simulink model "DCM_Test_v5"  (Simulink 7.5)
settings: Solver=FixedStepDiscrete  StartTime=0.0  StopTime=t(end)  FixedStep=SampleT  RelTol=1e-3
values from neighbouring files (symbols this model uses):
  apSampleTime = 0.01    [demoz2SlugsV5.m]
  R0 = single(Euler2DCMdeg( PHI_IC, THETA_IC, PSI_IC ))    [demoz2SlugsV5.m]
  SampleT = 0.02    [demoz2SlugsV5.m]
undefined symbols (not defined in the file or in its folder): DiscIntNeverNeededParam
libraries: simulink x11, dspmtrx3 x2
settings Model: Creator=Robert  LastModifiedBy=Robert
settings DataIOCC: LimitDataPoints=off

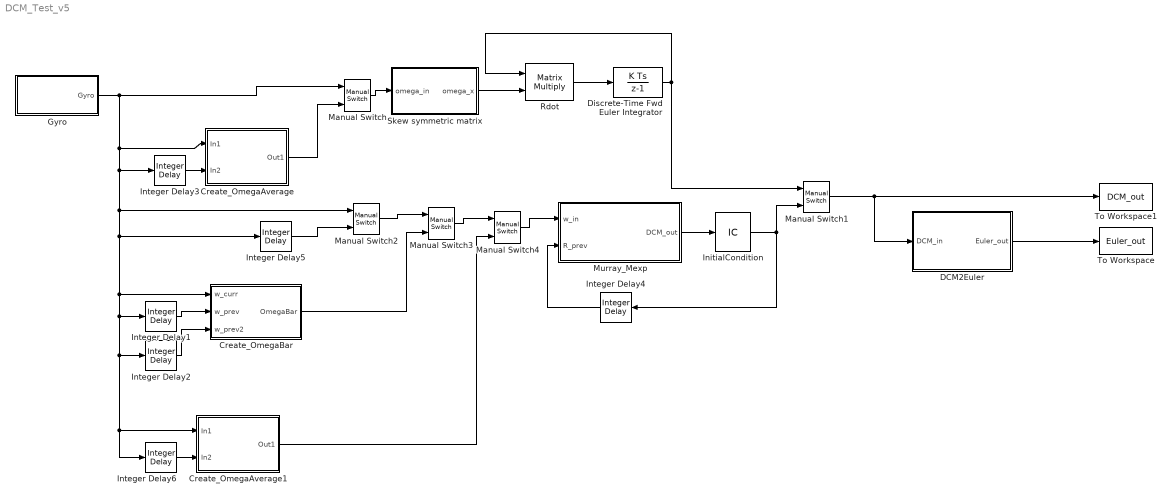
== system DCM_Test_v5 ==
  Create_OmegaAverage : Subsystem
  Create_OmegaAverage1 : Subsystem
  Create_OmegaBar : Subsystem
  DCM2Euler : Subsystem
  Discrete-Time Fwd Euler Integrator : DiscreteIntegrator  InitialCondition=R0  SampleTime=SampleT  OutDataTypeMode=single  OutDataType=fixdt(1, 16)  OutScaling=2^0  OutDataTypeStr=single  ICPrevOutput=DiscIntNeverNeededParam  ICPrevScaledInput=DiscIntNeverNeededParam
  Gyro : Subsystem
  InitialCondition : InitialCondition  Value=R0  SampleTime=apSampleTime
  Integer Delay{1,3..6} (5 alike) : simulink/Discrete/Integer Delay  vinit=0.0  samptime=-1  NumDelays=1
  Integer Delay2 : simulink/Discrete/Integer Delay  vinit=0.0  samptime=-1  NumDelays=2
  Manual Switch{,1..3} (4 alike) : simulink/Signal Routing/Manual Switch  SystemSampleTime=-1  sw=0  action=0  varsize=off
  Manual Switch4 : simulink/Signal Routing/Manual Switch  SystemSampleTime=-1  sw=1  action=0  varsize=off
  Murray_Mexp : Subsystem
  Rdot : Product  Multiplication=Matrix(*)  OutDataTypeMode=single  OutDataType=sfix(16)  OutScaling=2^0  OutDataTypeStr=single  SampleTime=SampleT
  Skew symmetric matrix : Subsystem
  To Workspace : ToWorkspace  VariableName=Euler_out  SampleTime=apSampleTime  SaveFormat=Structure
  To Workspace1 : ToWorkspace  VariableName=DCM_out  SampleTime=apSampleTime  SaveFormat=Structure
  wires:
  Discrete-Time Fwd Euler Integrator/1 -> Rdot/1, Manual Switch1/1
  DCM2Euler/1(Euler_out) -> To Workspace/1
  Rdot/1 -> Discrete-Time Fwd Euler Integrator/1
  Skew symmetric matrix/1(omega_x) -> Rdot/2
  Gyro/1(Gyro) -> Manual Switch/1, Create_OmegaAverage/1(In1), Integer Delay3/1, Create_OmegaBar/1(w_curr), Integer Delay1/1, Integer Delay2/1, Create_OmegaAverage1/1(In1), Integer Delay6/1, Integer Delay5/1, Manual Switch2/1
  Integer Delay3/1 -> Create_OmegaAverage/2(In2)
  Create_OmegaAverage/1(Out1) -> Manual Switch/2
  Manual Switch/1 -> Skew symmetric matrix/1(omega_in)
  Integer Delay2/1 -> Create_OmegaBar/3(w_prev2)
  Integer Delay1/1 -> Create_OmegaBar/2(w_prev)
  Create_OmegaBar/1(OmegaBar) -> Manual Switch3/2
  Murray_Mexp/1(DCM_out) -> InitialCondition/1
  Integer Delay4/1 -> Murray_Mexp/2(R_prev)
  InitialCondition/1 -> Integer Delay4/1, Manual Switch1/2
  Manual Switch1/1 -> To Workspace1/1, DCM2Euler/1(DCM_in)
  Integer Delay5/1 -> Manual Switch2/2
  Manual Switch2/1 -> Manual Switch3/1
  Integer Delay6/1 -> Create_OmegaAverage1/2(In2)
  Manual Switch3/1 -> Manual Switch4/1
  Manual Switch4/1 -> Murray_Mexp/1(w_in)
  Create_OmegaAverage1/1(Out1) -> Manual Switch4/2

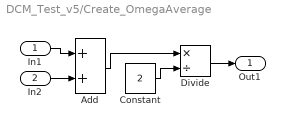
== system DCM_Test_v5/Create_OmegaAverage ==
  In1 : Inport
  In2 : Inport  Port=2
  Add : Sum  OutDataType=fixdt(1, 16)  OutScaling=2^-10
  Constant : Constant  Value=2  OutDataTypeMode=single  OutDataType=fixdt(1, 16)  OutScaling=2^0  OutDataTypeStr=single
  Divide : Product  Inputs=*/  OutDataType=fixdt(1, 16)  OutScaling=2^-10
  Out1 : Outport
  wires:
  Constant/1 -> Divide/2
  Add/1 -> Divide/1
  In1/1 -> Add/1
  In2/1 -> Add/2
  Divide/1 -> Out1/1

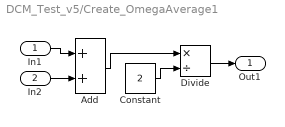
== system DCM_Test_v5/Create_OmegaAverage1 ==
  In1 : Inport
  In2 : Inport  Port=2
  Add : Sum  OutDataType=fixdt(1, 16)  OutScaling=2^-10
  Constant : Constant  Value=2  OutDataTypeMode=single  OutDataType=fixdt(1, 16)  OutScaling=2^0  OutDataTypeStr=single
  Divide : Product  Inputs=*/  OutDataType=fixdt(1, 16)  OutScaling=2^-10
  Out1 : Outport
  wires:
  Divide/1 -> Out1/1
  In2/1 -> Add/2
  In1/1 -> Add/1
  Add/1 -> Divide/1
  Constant/1 -> Divide/2

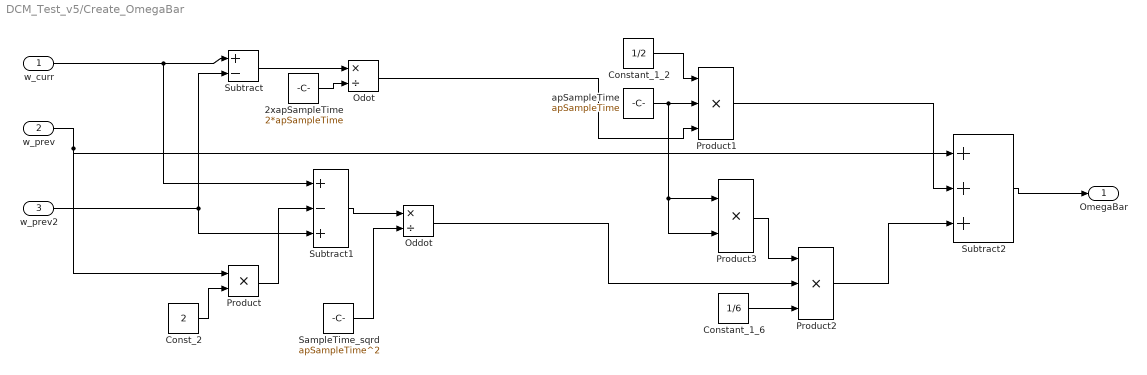
== system DCM_Test_v5/Create_OmegaBar ==
  w_curr : Inport
  w_prev : Inport  Port=2
  w_prev2 : Inport  Port=3
  2xapSampleTime : Constant  Value=2*apSampleTime  OutDataTypeMode=single  OutDataType=fixdt(1, 16)  OutScaling=2^0  OutDataTypeStr=single
  Const_2 : Constant  Value=2  OutDataTypeMode=single  OutDataType=fixdt(1, 16)  OutScaling=2^0  OutDataTypeStr=single
  Constant_1_2 : Constant  Value=1/2  OutDataTypeMode=single  OutDataType=fixdt(1, 16)  OutScaling=2^0  OutDataTypeStr=single
  Constant_1_6 : Constant  Value=1/6  OutDataTypeMode=single  OutDataType=fixdt(1, 16)  OutScaling=2^0  OutDataTypeStr=single
  Oddot : Product  Inputs=*/  OutDataType=fixdt(1, 16)  OutScaling=2^-10
  Odot : Product  Inputs=*/  OutDataType=fixdt(1, 16)  OutScaling=2^-10
  Product : Product  OutDataType=fixdt(1, 16)  OutScaling=2^0  RndMeth=Zero
  Product1 : Product  Inputs=3  OutDataType=fixdt(1, 16)  OutScaling=2^0  RndMeth=Zero
  Product2 : Product  Inputs=3  OutDataType=fixdt(1, 16)  OutScaling=2^0  RndMeth=Zero
  Product3 : Product  OutDataTypeMode=single  OutDataType=fixdt(1, 16)  OutScaling=2^0  OutDataTypeStr=single  SampleTime=apSampleTime  RndMeth=Zero
  SampleTime_sqrd : Constant  Value=apSampleTime^2  OutDataTypeMode=single  OutDataType=fixdt(1, 16)  OutScaling=2^0  OutDataTypeStr=single
  Subtract : Sum  Inputs=+-  OutDataType=fixdt(1, 16)  OutScaling=2^-10
  Subtract1 : Sum  Inputs=+-+  OutDataType=fixdt(1, 16)  OutScaling=2^-10
  Subtract2 : Sum  Inputs=+++  OutDataTypeMode=single  OutDataType=fixdt(1, 16)  OutScaling=2^-10  OutDataTypeStr=single
  apSampleTime : Constant  Value=apSampleTime  OutDataTypeMode=single  OutDataType=fixdt(1, 16)  OutScaling=2^0  OutDataTypeStr=single
  OmegaBar : Outport
  wires:
  Product2/1 -> Subtract2/3
  Oddot/1 -> Product2/2
  Product3/1 -> Product2/1
  Constant_1_6/1 -> Product2/3
  Product1/1 -> Subtract2/2
  Odot/1 -> Product1/3
  apSampleTime/1 -> Product3/2, Product3/1, Product1/2
  Constant_1_2/1 -> Product1/1
  Subtract2/1 -> OmegaBar/1
  Product/1 -> Subtract1/2
  Const_2/1 -> Product/2
  Subtract1/1 -> Oddot/1
  SampleTime_sqrd/1 -> Oddot/2
  2xapSampleTime/1 -> Odot/2
  Subtract/1 -> Odot/1
  w_prev2/1 -> Subtract1/3, Subtract/2
  w_curr/1 -> Subtract1/1, Subtract/1
  w_prev/1 -> Subtract2/1, Product/1

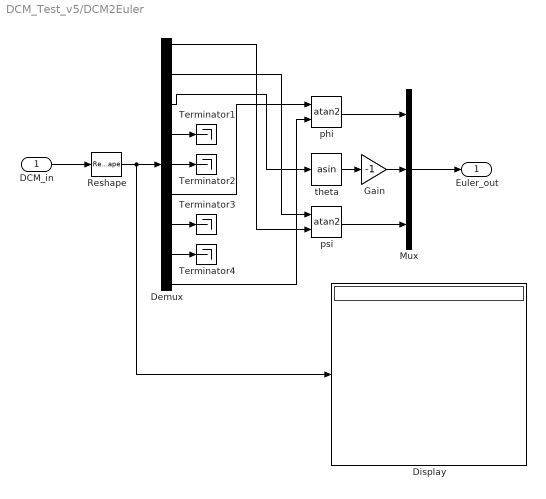
== system DCM_Test_v5/DCM2Euler ==
  DCM_in : Inport  OutDataType=fixdt(1, 16)  OutScaling=2^0
  Demux : Demux  Outputs=9
  Display : Display
  Gain : Gain  Gain=-1  ParameterDataType=fixdt(1, 16)  ParameterScaling=2^0  OutDataType=fixdt(1, 16)  OutScaling=2^0
  Mux : Mux  Inputs=3
  Reshape : Reshape
  Terminator{1..4} (4 alike) : Terminator
  phi : Trigonometry  Operator=atan2
  psi : Trigonometry  Operator=atan2
  theta : Trigonometry  Operator=asin
  Euler_out : Outport  OutDataType=fixdt(1, 16)  OutScaling=2^0
  wires:
  Demux/8 -> Terminator4/1
  Demux/7 -> Terminator3/1
  Demux/5 -> Terminator2/1
  Demux/4 -> Terminator1/1
  Demux/1 -> psi/2
  Demux/2 -> psi/1
  Demux/3 -> theta/1
  Demux/9 -> phi/2
  Demux/6 -> phi/1
  Gain/1 -> Mux/2
  Reshape/1 -> Display/1, Demux/1
  psi/1 -> Mux/3
  theta/1 -> Gain/1
  phi/1 -> Mux/1
  Mux/1 -> Euler_out/1
  DCM_in/1 -> Reshape/1

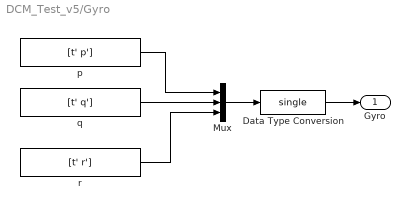
== system DCM_Test_v5/Gyro ==
  Data Type Conversion : DataTypeConversion  OutDataTypeMode=single  OutDataType=sfix(16)  OutScaling=2^0  OutDataTypeStr=single  SampleTime=SampleT
  Mux : Mux  Inputs=3
  p : FromWorkspace  VariableName=[t' p']  SampleTime=SampleT  Interpolate=off  OutputAfterFinalValue=Setting to zero
  q : FromWorkspace  VariableName=[t' q']  SampleTime=0.01  OutputAfterFinalValue=Setting to zero
  r : FromWorkspace  VariableName=[t' r']  SampleTime=0.01  OutputAfterFinalValue=Setting to zero
  Gyro : Outport  OutDataType=sfix(16)  OutScaling=2^0
  wires:
  Data Type Conversion/1 -> Gyro/1
  Mux/1 -> Data Type Conversion/1
  r/1 -> Mux/3
  q/1 -> Mux/2
  p/1 -> Mux/1

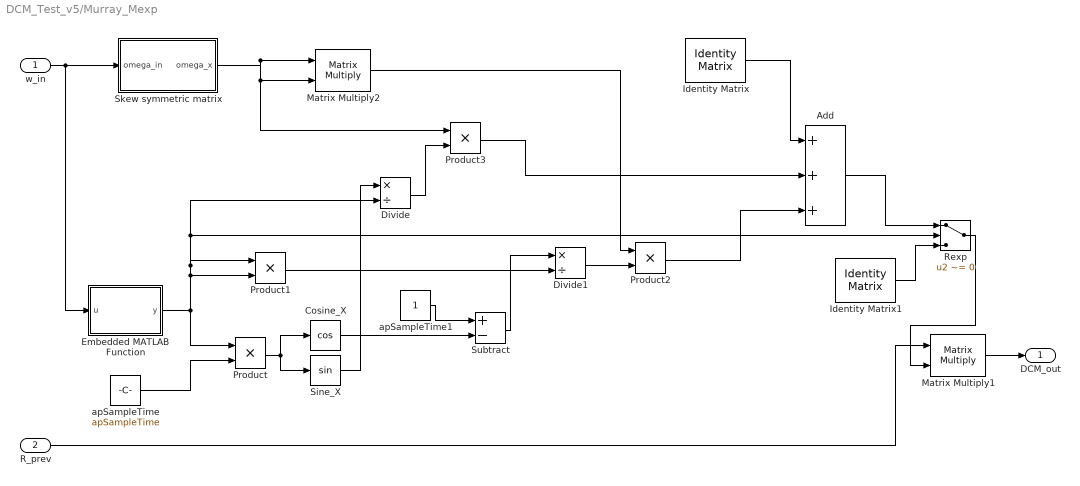
== system DCM_Test_v5/Murray_Mexp ==
  w_in : Inport  OutDataType=fixdt(1, 16)  OutScaling=2^0
  R_prev : Inport  Port=2  OutDataType=fixdt(1, 16)  OutScaling=2^0
  Add : Sum  Inputs=+++  OutDataTypeMode=single  OutDataType=fixdt(1, 16)  OutScaling=2^-10  OutDataTypeStr=single  SampleTime=apSampleTime
  Cosine_X : Trigonometry  Operator=cos
  Divide : Product  Inputs=*/  OutDataType=fixdt(1, 16)  OutScaling=2^-10
  Divide1 : Product  Inputs=*/  OutDataType=fixdt(1, 16)  OutScaling=2^-10
  Embedded MATLAB Function : Stateflow chart  TreatAsAtomicUnit=on
  Identity Matrix : dspmtrx3/Identity Matrix  Inherit=off  N=3  Ts=apSampleTime  dataType=single  isSigned=on  wordLen=16  udDataType=sfix(16)  fracBitsMode=Best precision  numFracBits=15
  Identity Matrix1 : dspmtrx3/Identity Matrix  Inherit=off  N=3  Ts=apSampleTime  dataType=single  isSigned=on  wordLen=16  udDataType=sfix(16)  fracBitsMode=Best precision  numFracBits=15
  Matrix Multiply1 : Product  Multiplication=Matrix(*)  OutDataType=sfix(16)  OutScaling=2^0
  Matrix Multiply2 : Product  Multiplication=Matrix(*)  OutDataType=sfix(16)  OutScaling=2^0
  Product{,1..3} (4 alike) : Product  OutDataType=fixdt(1, 16)  OutScaling=2^0  RndMeth=Zero
  Rexp : Switch  Criteria=u2 ~= 0  OutDataType=fixdt(1, 16)  OutScaling=2^0
  Sine_X : Trigonometry
  Skew symmetric matrix : Subsystem
  Subtract : Sum  Inputs=+-  OutDataType=fixdt(1, 16)  OutScaling=2^-10
  apSampleTime : Constant  Value=apSampleTime  OutDataTypeMode=single  OutDataType=fixdt(1, 16)  OutScaling=2^0  OutDataTypeStr=single
  apSampleTime1 : Constant  OutDataTypeMode=single  OutDataType=fixdt(1, 16)  OutScaling=2^0  OutDataTypeStr=single
  DCM_out : Outport  OutDataType=fixdt(1, 16)  OutScaling=2^0
  wires:
  Rexp/1 -> Matrix Multiply1/2
  Identity Matrix1/1 -> Rexp/3
  Add/1 -> Rexp/1
  Matrix Multiply1/1 -> DCM_out/1
  R_prev/1 -> Matrix Multiply1/1
  Product3/1 -> Add/2
  Divide/1 -> Product3/2
  Sine_X/1 -> Divide/1
  Product2/1 -> Add/3
  Matrix Multiply2/1 -> Product2/1
  Divide1/1 -> Product2/2
  Product1/1 -> Divide1/2
  Subtract/1 -> Divide1/1
  Cosine_X/1 -> Subtract/2
  apSampleTime1/1 -> Subtract/1
  Skew symmetric matrix/1(omega_x) -> Product3/1, Matrix Multiply2/2, Matrix Multiply2/1
  Product/1 -> Sine_X/1, Cosine_X/1
  apSampleTime/1 -> Product/2
  Embedded MATLAB Function/1(y) -> Rexp/2, Divide/2, Product1/1, Product1/2, Product/1
  Identity Matrix/1 -> Add/1
  w_in/1 -> Embedded MATLAB Function/1(u), Skew symmetric matrix/1(omega_in)

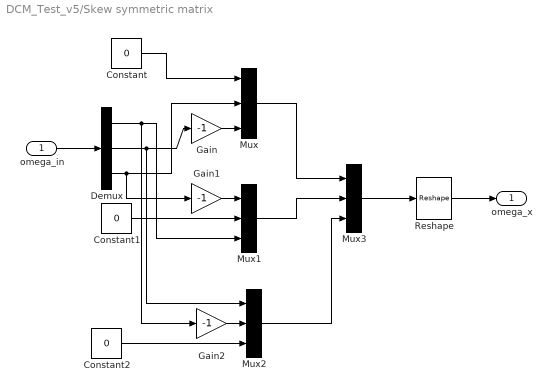
== system DCM_Test_v5/Skew symmetric matrix ==
  omega_in : Inport  PortDimensions=3  SampleTime=SampleT  OutDataType=fixdt(1, 16)  OutScaling=2^0
  Constant : Constant  Value=0  OutDataTypeMode=single  OutDataType=fixdt(1, 16)  OutScaling=2^0  OutDataTypeStr=single
  Constant1 : Constant  Value=0  OutDataTypeMode=single  OutDataType=fixdt(1, 16)  OutScaling=2^0  OutDataTypeStr=single
  Constant2 : Constant  Value=0  OutDataTypeMode=single  OutDataType=fixdt(1, 16)  OutScaling=2^0  OutDataTypeStr=single
  Demux : Demux  Outputs=3
  Gain : Gain  Gain=-1  ParameterDataType=fixdt(1, 16)  ParameterScaling=2^0  OutDataType=fixdt(1, 16)  OutScaling=2^0
  Gain1 : Gain  Gain=-1  ParameterDataType=fixdt(1, 16)  ParameterScaling=2^0  OutDataType=fixdt(1, 16)  OutScaling=2^0
  Gain2 : Gain  Gain=-1  ParameterDataType=fixdt(1, 16)  ParameterScaling=2^0  OutDataType=fixdt(1, 16)  OutScaling=2^0
  Mux{,1..3} (4 alike) : Mux  Inputs=3
  Reshape : Reshape  OutputDimensionality=Customize  OutputDimensions=[3,3]
  omega_x : Outport  PortDimensions=[3,3]  SampleTime=SampleT  OutDataType=fixdt(1, 16)  OutScaling=2^0
  wires:
  Gain2/1 -> Mux2/2
  Gain1/1 -> Mux1/1
  Gain/1 -> Mux/3
  Mux3/1 -> Reshape/1
  Mux2/1 -> Mux3/3
  Mux1/1 -> Mux3/2
  Mux/1 -> Mux3/1
  Constant2/1 -> Mux2/3
  Demux/1 -> Gain2/1, Mux1/3
  Constant1/1 -> Mux1/2
  Demux/2 -> Mux2/1, Gain/1
  Demux/3 -> Gain1/1, Mux/2
  Constant/1 -> Mux/1
  Reshape/1 -> omega_x/1
  omega_in/1 -> Demux/1

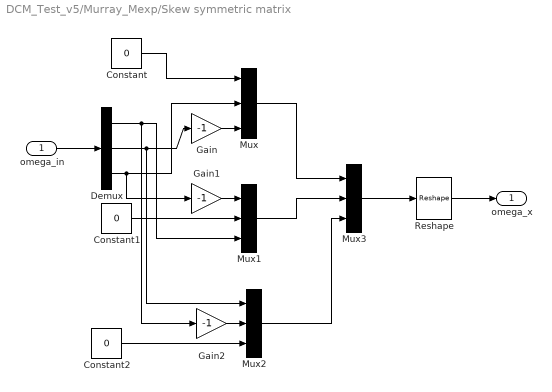
== system DCM_Test_v5/Murray_Mexp/Skew symmetric matrix ==
  omega_in : Inport  PortDimensions=3  SampleTime=SampleT  OutDataType=fixdt(1, 16)  OutScaling=2^0
  Constant : Constant  Value=0  OutDataTypeMode=single  OutDataType=fixdt(1, 16)  OutScaling=2^0  OutDataTypeStr=single
  Constant1 : Constant  Value=0  OutDataTypeMode=single  OutDataType=fixdt(1, 16)  OutScaling=2^0  OutDataTypeStr=single
  Constant2 : Constant  Value=0  OutDataTypeMode=single  OutDataType=fixdt(1, 16)  OutScaling=2^0  OutDataTypeStr=single
  Demux : Demux  Outputs=3
  Gain : Gain  Gain=-1  ParameterDataType=fixdt(1, 16)  ParameterScaling=2^0  OutDataType=fixdt(1, 16)  OutScaling=2^0
  Gain1 : Gain  Gain=-1  ParameterDataType=fixdt(1, 16)  ParameterScaling=2^0  OutDataType=fixdt(1, 16)  OutScaling=2^0
  Gain2 : Gain  Gain=-1  ParameterDataType=fixdt(1, 16)  ParameterScaling=2^0  OutDataType=fixdt(1, 16)  OutScaling=2^0
  Mux{,1..3} (4 alike) : Mux  Inputs=3
  Reshape : Reshape  OutputDimensionality=Customize  OutputDimensions=[3,3]
  omega_x : Outport  PortDimensions=[3,3]  SampleTime=SampleT  OutDataType=fixdt(1, 16)  OutScaling=2^0
  wires:
  omega_in/1 -> Demux/1
  Reshape/1 -> omega_x/1
  Constant/1 -> Mux/1
  Demux/3 -> Mux/2, Gain1/1
  Demux/2 -> Gain/1, Mux2/1
  Constant1/1 -> Mux1/2
  Demux/1 -> Mux1/3, Gain2/1
  Constant2/1 -> Mux2/3
  Mux/1 -> Mux3/1
  Mux1/1 -> Mux3/2
  Mux2/1 -> Mux3/3
  Mux3/1 -> Reshape/1
  Gain/1 -> Mux/3
  Gain1/1 -> Mux1/1
  Gain2/1 -> Mux2/2

== matlab function Murray_Mexp/Embedded MATLAB Function ==
  data: u input double; y output double
function y = GetNorm(u)
%#eml
% Function returns the 2-norm of the input argument.

y = norm(u);
